simulink model "SIMULATION FILE"  (R2024a)
settings: Solver=VariableStepAuto  StartTime=0.0  StopTime=10  RelTol=1e-3
libraries: spspowerguiLib x1
settings Model: Creator=DELL  LastModifiedBy=plali

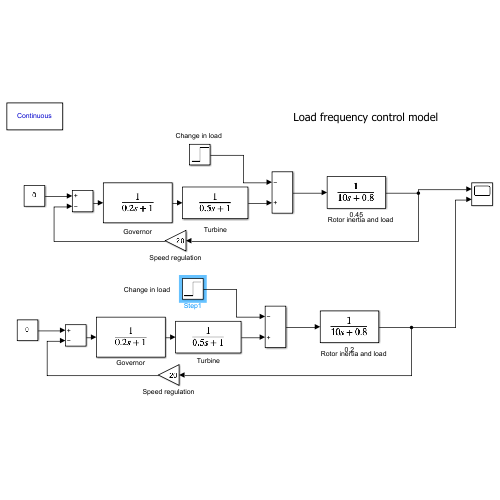
[thumbnail: Simulink's stored preview of the top-level diagram]
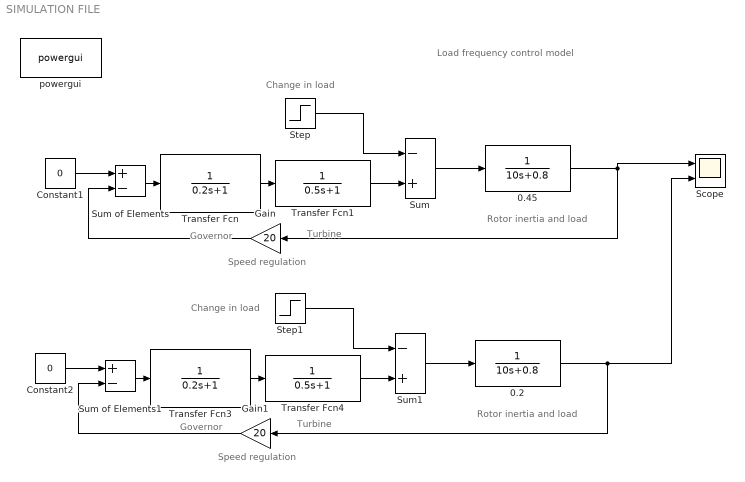
== system SIMULATION FILE ==
  note: Load frequency control model
  note: Speed regulation
  note: Rotor inertia and load
  note: Turbine
  note: Governor
  note: Change in load
  note: Turbine
  note: Change in load
  note: Speed regulation
  note: Governor
  note: Rotor inertia and load
  0.2 : TransferFcn  Denominator=[10 0.8]
  0.45 : TransferFcn  Denominator=[10 0.8]
  Constant1 : Constant  Value=0
  Constant2 : Constant  Value=0
  Gain : Gain  Gain=20
  Gain1 : Gain  Gain=20
  Scope : Scope  NumInputPorts=2
  Step : Step  After=0.45  SampleTime=0
  Step1 : Step  After=0.2  SampleTime=0
  Sum : Sum  Inputs=-+
  Sum of Elements : Sum  Inputs=+-
  Sum of Elements1 : Sum  Inputs=+-
  Sum1 : Sum  Inputs=-+
  Transfer Fcn : TransferFcn  Denominator=[0.2 1]
  Transfer Fcn1 : TransferFcn  Denominator=[0.5 1]
  Transfer Fcn3 : TransferFcn  Denominator=[0.2 1]
  Transfer Fcn4 : TransferFcn  Denominator=[0.5 1]
  powergui : spspowerguiLib/powergui  Priority=1  SimulationMode=Continuous  SampleTime=50e-6  frequency=60  Iterations=50  frequencyindice=60  Pbase=100e6  ErrMax=1e-4  UnitsV=kV  UnitsW=MW  buscounter=0  FunctionMessages=off  echomessages=off  EnableUseOfTLC=off  CurrentSourceSwitches=off  DisableSnubberDevices=off  DisableRonSwitches=off  DisableVfSwitches=off  DisplayEquations=off  AutomaticDiscreteSolvers=off  SolverType=Tustin/Backward Euler (TBE)  Interpol=off  ExternalGateDelay=off  methode=off  Ts=100  x0status=blocks  SPID=on  SwTol=0  HookPort=off  NonlinearTolerance=1e-4  nMaxIteration=100  ContinueOnMaxIteration=off  RestoreLinks=warning  ResistiveCurrentMeasurement=off  Frange=[0:2:500]  Ylog=off  Xlog=on  ShowGrid=off  save=off  variable=ZData  structure=0  ZoomFFT=off  StartTime=0.0  cycles=1  DisplayStyle=1  fundamental=60  FreqAxis=off  MaxFrequency=1000  frequencyindicesteady=1  RmsSteady=1  display=off
  wires:
  0.45/1 -> Scope/1, Gain/1
  Sum/1 -> 0.45/1
  Transfer Fcn/1 -> Transfer Fcn1/1
  Gain/1 -> Sum of Elements/2
  Step/1 -> Sum/1
  Transfer Fcn1/1 -> Sum/2
  Sum of Elements/1 -> Transfer Fcn/1
  Constant1/1 -> Sum of Elements/1
  Gain1/1 -> Sum of Elements1/2
  Transfer Fcn4/1 -> Sum1/2
  Sum of Elements1/1 -> Transfer Fcn3/1
  Transfer Fcn3/1 -> Transfer Fcn4/1
  0.2/1 -> Scope/2, Gain1/1
  Sum1/1 -> 0.2/1
  Step1/1 -> Sum1/1
  Constant2/1 -> Sum of Elements1/1
